simulink model "Full_Polyphase_System"  (R2025b)
settings: Solver=VariableStepAuto  StartTime=0.0  StopTime=10.0  RelTol=1e-3
values from neighbouring files (symbols this model uses):
  E0_bpf1 = h_bpf1(1:3:end)    [main.m]
  E0_bpf2 = h_bpf2(1:3:end)    [main.m]
  E0_lpf = h_lpf(1:3:end)    [main.m]
  E1_bpf1 = h_bpf1(2:3:end)    [main.m]
  E1_bpf2 = h_bpf2(2:3:end)    [main.m]
  E1_lpf = h_lpf(2:3:end)    [main.m]
  E2_bpf1 = h_bpf1(3:3:end)    [main.m]
  E2_bpf2 = h_bpf2(3:3:end)    [main.m]
  E2_lpf = h_lpf(3:3:end)    [main.m]
undefined symbols (not defined in the file or in its folder): dspblkCoreblockFVToolHelper, gcbh
libraries: dspsigops x5
settings Model: Creator=jai-raj  LastModifiedBy=jai-raj

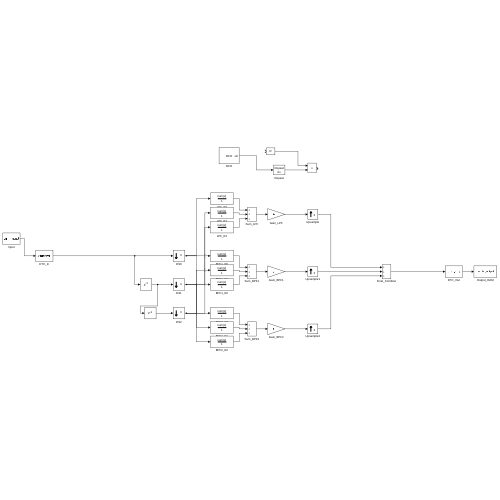
[thumbnail: Simulink's stored preview of the top-level diagram]
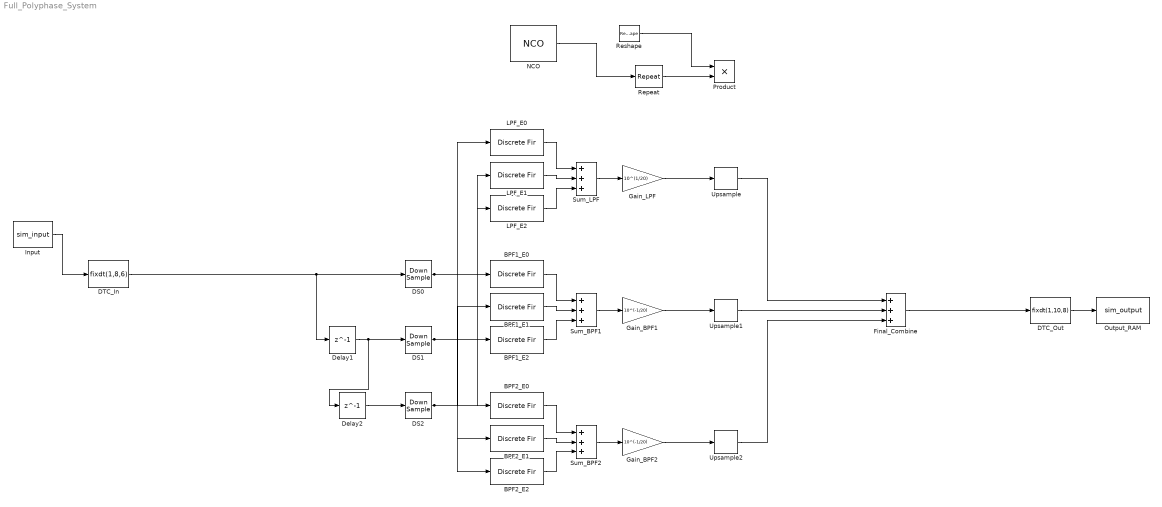
== system Full_Polyphase_System ==
  BPF1_E0 : DiscreteFir  LoadFcn=dspblkCoreblockFVToolHelper(gcbh,'load');  Coefficients=E0_bpf1
      settings: CopyFcn=dspblkCoreblockFVToolHelper(gcbh,'copy');  DeleteFcn=dspblkCoreblockFVToolHelper(gcbh,'close');  ModelCloseFcn=dspblkCoreblockFVToolHelper(gcbh,'close');  PreSaveFcn=dspblkCoreblockFVToolHelper(gcbh,'presave');  PostSaveFcn=dspblkCoreblockFVToolHelper(gcbh,'postsave');  CloseFcn=dspblkCoreblockFVToolHelper(gcbh,'close');
  BPF1_E1 : DiscreteFir  Coefficients=E1_bpf1
  BPF1_E2 : DiscreteFir  LoadFcn=dspblkCoreblockFVToolHelper(gcbh,'load');  Coefficients=E2_bpf1
      settings: CopyFcn=dspblkCoreblockFVToolHelper(gcbh,'copy');  DeleteFcn=dspblkCoreblockFVToolHelper(gcbh,'close');  ModelCloseFcn=dspblkCoreblockFVToolHelper(gcbh,'close');  PreSaveFcn=dspblkCoreblockFVToolHelper(gcbh,'presave');  PostSaveFcn=dspblkCoreblockFVToolHelper(gcbh,'postsave');  CloseFcn=dspblkCoreblockFVToolHelper(gcbh,'close');
  BPF2_E0 : DiscreteFir  Coefficients=E0_bpf2
  BPF2_E1 : DiscreteFir  Coefficients=E1_bpf2
  BPF2_E2 : DiscreteFir  Coefficients=E2_bpf2
  DS0 : DownSample  N=3  AllowArbitraryFixedInput=on
  DS1 : DownSample  N=3  AllowArbitraryFixedInput=on
  DS2 : DownSample  N=3  AllowArbitraryFixedInput=on
  DTC_In : DataTypeConversion  OutDataTypeStr=fixdt(1,8,6)  SaturateOnIntegerOverflow=off  RndMeth=Floor
  DTC_Out : DataTypeConversion  OutDataTypeStr=fixdt(1,10,8)  SaturateOnIntegerOverflow=off  RndMeth=Floor
  Delay1 : Delay  DelayLength=1
  Delay2 : Delay  DelayLength=1
  Final_Combine : Sum  Inputs=+++
  Gain_BPF1 : Gain  Gain=10^(-1/20)
  Gain_BPF2 : Gain  Gain=10^(-1/20)
  Gain_LPF : Gain  Gain=10^(1/20)
  Input : FromWorkspace  VariableName=sim_input
  LPF_E0 : DiscreteFir  LoadFcn=dspblkCoreblockFVToolHelper(gcbh,'load');  Coefficients=E0_lpf
      settings: CopyFcn=dspblkCoreblockFVToolHelper(gcbh,'copy');  DeleteFcn=dspblkCoreblockFVToolHelper(gcbh,'close');  ModelCloseFcn=dspblkCoreblockFVToolHelper(gcbh,'close');  PreSaveFcn=dspblkCoreblockFVToolHelper(gcbh,'presave');  PostSaveFcn=dspblkCoreblockFVToolHelper(gcbh,'postsave');  CloseFcn=dspblkCoreblockFVToolHelper(gcbh,'close');
  LPF_E1 : DiscreteFir  Coefficients=E1_lpf
  LPF_E2 : DiscreteFir  LoadFcn=dspblkCoreblockFVToolHelper(gcbh,'load');  Coefficients=E2_lpf
      settings: CopyFcn=dspblkCoreblockFVToolHelper(gcbh,'copy');  DeleteFcn=dspblkCoreblockFVToolHelper(gcbh,'close');  ModelCloseFcn=dspblkCoreblockFVToolHelper(gcbh,'close');  PreSaveFcn=dspblkCoreblockFVToolHelper(gcbh,'presave');  PostSaveFcn=dspblkCoreblockFVToolHelper(gcbh,'postsave');  CloseFcn=dspblkCoreblockFVToolHelper(gcbh,'close');
  NCO : dspsigops/NCO  AccIncSrc=Specify via dialog  AccInc=751619276  PhaseOffsetSrc=Specify via dialog  PhaseOffset=0  AccumWL=32  HasDither=on  DitherWL=4  PNgeneratorLength=19  HasPhaseQuantizer=on  TableDepth=12  HasOutputPhaseError=off  Formula=Sine  DataType=double  OutputWL=16  OutputFL=14  CompMethod=Table lookup (no interpolation)  SampleTime=1  SamplesPerFrame=8  OutputFrames=off
      settings: LibrarySourceBlock=dspsrcs4/NCO
  Output_RAM : ToWorkspace  VariableName=sim_output  SaveFormat=Timeseries  SampleTime=-1
  Product : Product
  Repeat : dspsigops/Repeat  FactorSource=Dialog parameter  N=6  Nmax=16  InputProcessing=Columns as channels (frame based)  RateOptions=Enforce single-rate processing  ic=0  mode=Unused parameter value
      settings: LibrarySourceBlock=dsphdlsupportsigops/Repeat
  Reshape : Reshape  OutputDimensionality=Customize  OutputDimensions=[8,6]
  Sum_BPF1 : Sum  Inputs=+++
  Sum_BPF2 : Sum  Inputs=+++
  Sum_LPF : Sum  Inputs=+++
  Upsample : dspsigops/Upsample  FactorSource=Dialog parameter  N=3  Nmax=16  phase=0  RateOptions=Allow multirate processing  ic=0  mode=Unused parameter value
      settings: LibrarySourceBlock=dsphdlsupportsigops/Upsample
  Upsample1 : dspsigops/Upsample  FactorSource=Dialog parameter  N=3  Nmax=16  phase=0  RateOptions=Allow multirate processing  ic=0  mode=Unused parameter value
      settings: LibrarySourceBlock=dsphdlsupportsigops/Upsample
  Upsample2 : dspsigops/Upsample  FactorSource=Dialog parameter  N=3  Nmax=16  phase=0  RateOptions=Allow multirate processing  ic=0  mode=Unused parameter value
      settings: LibrarySourceBlock=dsphdlsupportsigops/Upsample
  wires:
  Input/1 -> DTC_In/1
  DTC_In/1 -> Delay1/1, DS0/1
  Delay1/1 -> Delay2/1, DS1/1
  Delay2/1 -> DS2/1
  DS0/1 -> LPF_E0/1, BPF1_E0/1, BPF2_E0/1
  DS1/1 -> LPF_E1/1, BPF1_E1/1, BPF2_E1/1
  DS2/1 -> LPF_E2/1, BPF1_E2/1, BPF2_E2/1
  LPF_E0/1 -> Sum_LPF/1
  LPF_E1/1 -> Sum_LPF/2
  LPF_E2/1 -> Sum_LPF/3
  Sum_LPF/1 -> Gain_LPF/1
  BPF1_E0/1 -> Sum_BPF1/1
  BPF1_E1/1 -> Sum_BPF1/2
  BPF1_E2/1 -> Sum_BPF1/3
  Sum_BPF1/1 -> Gain_BPF1/1
  BPF2_E0/1 -> Sum_BPF2/1
  BPF2_E1/1 -> Sum_BPF2/2
  BPF2_E2/1 -> Sum_BPF2/3
  Sum_BPF2/1 -> Gain_BPF2/1
  Gain_LPF/1 -> Upsample/1
  Gain_BPF1/1 -> Upsample1/1
  Gain_BPF2/1 -> Upsample2/1
  Final_Combine/1 -> DTC_Out/1
  DTC_Out/1 -> Output_RAM/1
  NCO/1 -> Repeat/1
  Reshape/1 -> Product/1
  Repeat/1 -> Product/2
  Upsample2/1 -> Final_Combine/3
  Upsample1/1 -> Final_Combine/2
  Upsample/1 -> Final_Combine/1
